simulink model "feedbacksInGuyton72"  (R2018a)
settings: Solver=VariableStepAuto  StartTime=0.0  StopTime=inf  RelTol=1e-3
settings Model: Creator=Jirka  LastModifiedBy=Jirka

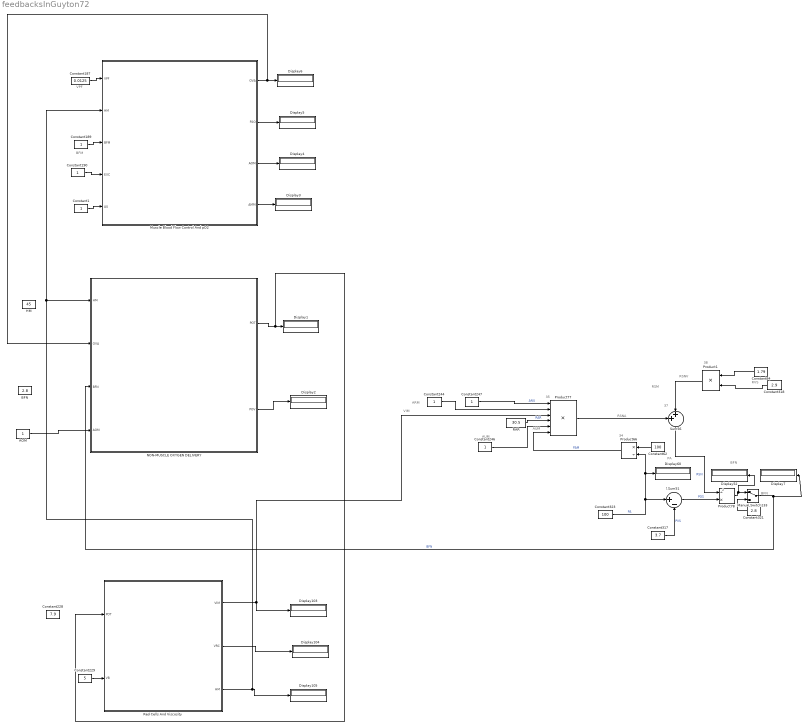
== system feedbacksInGuyton72 ==
  note: VPF
  note: BFM
  note: AUM
  note: ARM
  note: BFN
  note: VIM
  note: AUM
  note: RSM
  note: 1
  note: 35
  note: RSNV
  note: 37
  note: 2
  note: BFN
  note: PA
  note: 34
  note: RSNA
  note: RVS
  note: 38
  AOM : Constant
  BFN : Constant  Value=2.8
  Constant{1,189..190,244,246..247} (6 alike) : Constant
  Constant187 : Constant  Value=0.0125
  Constant228 : Constant  Value=7.9
  Constant229 : Constant  Value=5
  Constant317 : Constant  Value=3.7
  Constant318 : Constant  Value=2.9
  Constant321 : Constant  Value=2.8
  Constant323 : Constant  Value=100
  Constant62 : Constant  Value=100
  Constant84 : Constant  Value=1.79
  Display{1..7,52,60,103..105} (12 alike) : Display
  HM : Constant  Value=45
  Manual Switch133 : ManualSwitch
  Muscle Blood Flow Control And pO2 : Subsystem
      settings: MinAlgLoopOccurrences=on
      mask Display: disp('MUSCLE BLOOD FLOW CONTROL AND PO2\n\nINTPUTS:\nVPF - volume of free fluid in the pulmonary interstitium \nHM - hematocrit [%]\nBFM - blood flow in muscles \n [l/min]\nEXC - Effect of excercise on the metabolic usage \nof oxygen by the muscles [ratio to resting state]\nAU - overall activity of autonomic system\n  \nOUTPUTS:\nOVA - oxygen content of arterial blood \n[ml O2 STPD/l blood] \nP2O - muscle cell PO2  [torr]\nAOM - autonomic effect on tissue oxygenation \nAMM - muscle vascular constriction caused by logical tissue control\n[multiplifier, ratio to normal]\n\n')
  NON-MUSCLE OXYGEN DELIVERY : Subsystem
      mask Display: disp('NON-MUSCLE OXYGEN DELIVERY\n\nINTPUTS:\nHM-hematocrit [%]\nOVA-oxygen volume in aortic blood [ml O2/l blood]\nBFN-blood flow in non-muscle, non-renal tissues [l/min]\nAOM-autonomic effect on tissue oxygen utilization\n\nOUTPUTS:\nPOT-non-muscle cell PO2  [torr]\nPOV-non-muscle venous PO2 [torr]\n')
  Product1 : Product  SaturateOnIntegerOverflow=on  RndMeth=Zero  InputSameDT=on  OutDataTypeStr=Inherit: Same as first input
  Product66 : Product  Inputs=*/  SaturateOnIntegerOverflow=on  RndMeth=Zero  InputSameDT=on  OutDataTypeStr=Inherit: Same as first input
  Product77 : Product  Inputs=6  SaturateOnIntegerOverflow=on  RndMeth=Zero  InputSameDT=on  OutDataTypeStr=Inherit: Same as first input
  Product78 : Product  Inputs=/*  SaturateOnIntegerOverflow=on  RndMeth=Zero  InputSameDT=on  OutDataTypeStr=Inherit: Same as first input
  RAR : Constant  Value=30.5
  Red Cells And Viscosity : Subsystem
      settings: MinAlgLoopOccurrences=on
      mask Display: disp('RED CELLS AND VISCOSITY\n\nINTPUT:\nPOT - non-muscle cell PO2 [torr]\nVB - volume of blood [l]\n\nOUTPUT:\nVIM - blood viscosity [ratio to normal]\nHM - hematocrit [%]\nVRC - volume of red blood cells []\n')
  Sum51 : Sum  Inputs=|+-  SaturateOnIntegerOverflow=on  InputSameDT=on  OutDataTypeStr=Inherit: Same as first input
  Sum56 : Sum  Inputs=++|  SaturateOnIntegerOverflow=on  InputSameDT=on  OutDataTypeStr=Inherit: Same as first input
  wires:
  Constant229/1 -> Red Cells And Viscosity/2(VB)
  Red Cells And Viscosity/2(VRC) -> Display104/1
  AOM/1 -> NON-MUSCLE OXYGEN DELIVERY/4(AOM)
  NON-MUSCLE OXYGEN DELIVERY/2(POV) -> Display2/1
  Muscle Blood Flow Control And pO2/2(P2O) -> Display5/1
  Muscle Blood Flow Control And pO2/3(AOM) -> Display4/1
  Muscle Blood Flow Control And pO2/4(AMM) -> Display3/1
  Constant190/1 -> Muscle Blood Flow Control And pO2/4(EXC)
  Constant189/1 -> Muscle Blood Flow Control And pO2/3(BFM)
  Constant187/1 -> Muscle Blood Flow Control And pO2/1(VPF)
  Constant1/1 -> Muscle Blood Flow Control And pO2/5(AU)
  Muscle Blood Flow Control And pO2/1(OVA) -> NON-MUSCLE OXYGEN DELIVERY/2(OVA), Display6/1
  NON-MUSCLE OXYGEN DELIVERY/1(POT) -> Red Cells And Viscosity/1(POT), Display1/1
  Red Cells And Viscosity/3(HM) -> Muscle Blood Flow Control And pO2/2(HM), NON-MUSCLE OXYGEN DELIVERY/1(HM), Display105/1
  Sum56/1 -> Product78/1  "RSN"
  Red Cells And Viscosity/1(VIM) -> Display103/1, Product77/3
  Constant247/1 -> Product77/1  "ANU"
  Product1/1 -> Sum56/2
  Manual Switch133/1 -> Display7/1, NON-MUSCLE OXYGEN DELIVERY/3(BFN)  "BFN"
  Sum51/1 -> Product78/2  "PGS"
  Product66/1 -> Product77/6  "PAM"
  Constant62/1 -> Product66/1
  Product77/1 -> Sum56/1
  Constant246/1 -> Product77/5
  Constant244/1 -> Product77/2
  Constant323/1 -> Sum51/1, Display60/1, Product66/2  "PA"
  RAR/1 -> Product77/4  "RAR"
  Constant321/1 -> Manual Switch133/2
  Product78/1 -> Display52/1, Manual Switch133/1
  Constant84/1 -> Product1/1
  Constant318/1 -> Product1/2
  Constant317/1 -> Sum51/2  "PVS"

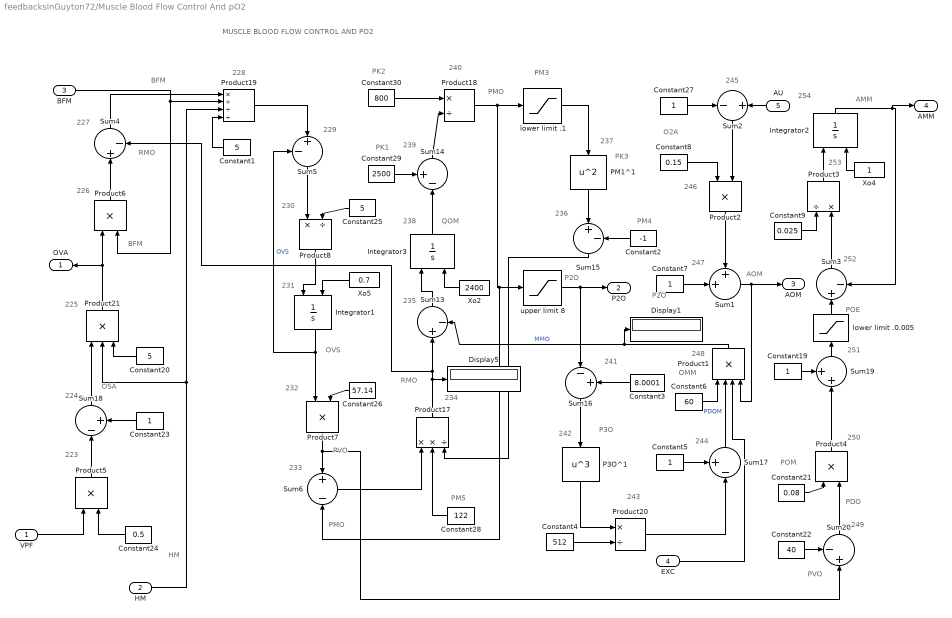
== system feedbacksInGuyton72/Muscle Blood Flow Control And pO2 ==
  note: PM5
  note: POM
  note: 244
  note: AMM
  note: 249
  note: PM3
  note: POE
  note: PK1
  note: RMO
  note: 251
  note: 236
  note: 254
  note: 240
  note: 245
  note: P2O
  note: 250
  note: P2O
  note: 252
  note: PMO
  note: OSA
  note: 253
  note: PM4
  note: PDO
  note: 247
  note: 237
  note: 239
  note: PK3
  note: PMO
  note: 246
  note: RMO
  note: BFM
  note: 243
  note: 242
  note: BFM
  note: PVO
  note: HM
  note: AOM
  note: OMM
  note: MUSCLE BLOOD FLOW CONTROL AND PO2
  note: 223
  note: 229
  note: 235
  note: 232
  note: O2A
  note: 227
  note: QOM
  note: 241
  note: PVO
  note: 228
  note: 248
  note: 226
  note: 225
  note: 231
  note: OVS
  note: 230
  note: 238
  note: P3O
  note: 234
  note: 224
  note: 233
  note: PK2
  VPF : Inport
  HM : Inport  Port=2
  BFM : Inport  Port=3
  EXC : Inport  Port=4
  AU : Inport  Port=5
  Constant1 : Constant  Value=5
  Constant{5,7,19,23,27} (5 alike) : Constant
  Constant2 : Constant  Value=-1
  Constant20 : Constant  Value=5
  Constant21 : Constant  Value=0.08
  Constant22 : Constant  Value=40
  Constant24 : Constant  Value=0.5
  Constant25 : Constant  Value=5
  Constant26 : Constant  Value=57.14
  Constant28 : Constant  Value=122
  Constant29 : Constant  Value=2500
  Constant3 : Constant  Value=8.0001
  Constant30 : Constant  Value=800
  Constant4 : Constant  Value=512
  Constant6 : Constant  Value=60
  Constant8 : Constant  Value=0.15
  Constant9 : Constant  Value=0.025
  Display1 : Display
  Display5 : Display
  Integrator1 : Integrator  InitialConditionSource=external
  Integrator2 : Integrator  InitialConditionSource=external  InitialCondition=2399.9633789
  Integrator3 : Integrator  InitialConditionSource=external  InitialCondition=2399.9633789
  P3O^1 : Fcn  Expr=u^3
  PM1^1 : Fcn  Expr=u^2
  Product1 : Product  Inputs=4  SaturateOnIntegerOverflow=on  RndMeth=Zero  InputSameDT=on  OutDataTypeStr=Inherit: Same as first input
  Product17 : Product  Inputs=**/  SaturateOnIntegerOverflow=on  RndMeth=Zero  InputSameDT=on  OutDataTypeStr=Inherit: Same as first input
  Product18 : Product  Inputs=*/  SaturateOnIntegerOverflow=on  RndMeth=Zero  InputSameDT=on  OutDataTypeStr=Inherit: Same as first input
  Product19 : Product  Inputs=*///  SaturateOnIntegerOverflow=on  RndMeth=Zero  InputSameDT=on  OutDataTypeStr=Inherit: Same as first input
  Product{2,4..7} (5 alike) : Product  SaturateOnIntegerOverflow=on  RndMeth=Zero  InputSameDT=on  OutDataTypeStr=Inherit: Same as first input
  Product20 : Product  Inputs=*/  SaturateOnIntegerOverflow=on  RndMeth=Zero  InputSameDT=on  OutDataTypeStr=Inherit: Same as first input
  Product21 : Product  Inputs=3  SaturateOnIntegerOverflow=on  RndMeth=Zero  InputSameDT=on  OutDataTypeStr=Inherit: Same as first input
  Product3 : Product  Inputs=/*  SaturateOnIntegerOverflow=on  RndMeth=Zero  InputSameDT=on  OutDataTypeStr=Inherit: Same as first input
  Product8 : Product  Inputs=*/  SaturateOnIntegerOverflow=on  RndMeth=Zero  InputSameDT=on  OutDataTypeStr=Inherit: Same as first input
  Sum1 : Sum  Inputs=++|  SaturateOnIntegerOverflow=on  InputSameDT=on  OutDataTypeStr=Inherit: Same as first input
  Sum{3..4,13,15} (4 alike) : Sum  Inputs=|+-  SaturateOnIntegerOverflow=on  InputSameDT=on  OutDataTypeStr=Inherit: Same as first input
  Sum14 : Sum  Inputs=+-|  SaturateOnIntegerOverflow=on  InputSameDT=on  OutDataTypeStr=Inherit: Same as first input
  Sum16 : Sum  Inputs=|-+  SaturateOnIntegerOverflow=on  InputSameDT=on  OutDataTypeStr=Inherit: Same as first input
  Sum17 : Sum  Inputs=+-|  SaturateOnIntegerOverflow=on  InputSameDT=on  OutDataTypeStr=Inherit: Same as first input
  Sum18 : Sum  Inputs=|-+  SaturateOnIntegerOverflow=on  InputSameDT=on  OutDataTypeStr=Inherit: Same as first input
  Sum19 : Sum  Inputs=++|  SaturateOnIntegerOverflow=on  InputSameDT=on  OutDataTypeStr=Inherit: Same as first input
  Sum2 : Sum  Inputs=-|+  SaturateOnIntegerOverflow=on  InputSameDT=on  OutDataTypeStr=Inherit: Same as first input
  Sum20 : Sum  Inputs=-+|  SaturateOnIntegerOverflow=on  InputSameDT=on  OutDataTypeStr=Inherit: Same as first input
  Sum5 : Sum  Inputs=-+|  SaturateOnIntegerOverflow=on  InputSameDT=on  OutDataTypeStr=Inherit: Same as first input
  Sum6 : Sum  Inputs=+|-  SaturateOnIntegerOverflow=on  InputSameDT=on  OutDataTypeStr=Inherit: Same as first input
  Xo2 : Constant  Value=2400  VectorParams1D=off
  Xo4 : Constant  VectorParams1D=off
  Xo5 : Constant  Value=0.7  VectorParams1D=off
  lower limit .0.005 : Saturate  UpperLimit=inf  LowerLimit=0.005  LinearizeAsGain=off
  lower limit .1 : Saturate  UpperLimit=inf  LowerLimit=0.001  LinearizeAsGain=off
  "upper limit 8 " : Saturate  UpperLimit=8  LowerLimit=0  LinearizeAsGain=off
  OVA : Outport
  P2O : Outport  Port=2
  AOM : Outport  Port=3
  AMM : Outport  Port=4
  wires:
  Constant1/1 -> Product19/4
  PM1^1/1 -> Sum15/1
  Product2/1 -> Sum1/1
  Integrator2/1 -> AMM/1, Sum3/2
  Sum13/1 -> Integrator3/1
  Constant4/1 -> Product20/2
  Constant28/1 -> Product17/2
  Constant25/1 -> Product8/2
  Sum17/1 -> Product1/2  "PDOM"
  Product1/1 -> Display1/1, Sum13/2  "MMO"
  Product5/1 -> Sum18/1
  Constant27/1 -> Sum2/1
  Constant2/1 -> Sum15/2
  Sum16/1 -> P3O^1/1
  Constant29/1 -> Sum14/1
  Product21/1 -> OVA/1, Product6/1
  Sum20/1 -> Product4/2
  Constant24/1 -> Product5/2
  Xo4/1 -> Integrator2/2
  Constant21/1 -> Product4/1
  Constant30/1 -> Product18/1
  Xo2/1 -> Integrator3/2
  Sum15/1 -> Product17/3
  lower limit .0.005/1 -> Sum3/1
  Constant8/1 -> Product2/1
  Product4/1 -> Sum19/2
  Constant19/1 -> Sum19/1
  P3O^1/1 -> Product20/1
  Product18/1 -> lower limit .1/1, Sum6/2, "upper limit 8 "/1
  Sum2/1 -> Product2/2
  Product17/1 -> Display5/1, Sum4/2, Sum13/1
  Constant3/1 -> Sum16/2
  Product20/1 -> Sum17/2
  Constant9/1 -> Product3/1
  Constant6/1 -> Product1/1
  Constant5/1 -> Sum17/1
  Sum3/1 -> Product3/2
  Integrator3/1 -> Sum14/2
  Product3/1 -> Integrator2/1
  Sum5/1 -> Product8/1
  Product19/1 -> Sum5/2
  Sum1/1 -> AOM/1, Product1/4
  Constant26/1 -> Product7/2
  Sum6/1 -> Product17/1
  Product7/1 -> Sum6/1, Sum20/2
  Sum18/1 -> Product21/1
  Xo5/1 -> Integrator1/2
  Product8/1 -> Integrator1/1
  Sum14/1 -> Product18/2
  Integrator1/1 -> Sum5/1, Product7/1  "OVS"
  Constant7/1 -> Sum1/2
  Constant23/1 -> Sum18/2
  Product6/1 -> Sum4/1
  lower limit .1/1 -> PM1^1/1
  Constant22/1 -> Sum20/1
  "upper limit 8 "/1 -> P2O/1, Sum16/1
  Sum19/1 -> lower limit .0.005/1
  Sum4/1 -> Product19/1
  Constant20/1 -> Product21/3
  VPF/1 -> Product5/1
  EXC/1 -> Product1/3
  AU/1 -> Sum2/2
  BFM/1 -> Product6/2, Product19/2
  HM/1 -> Product19/3, Product21/2

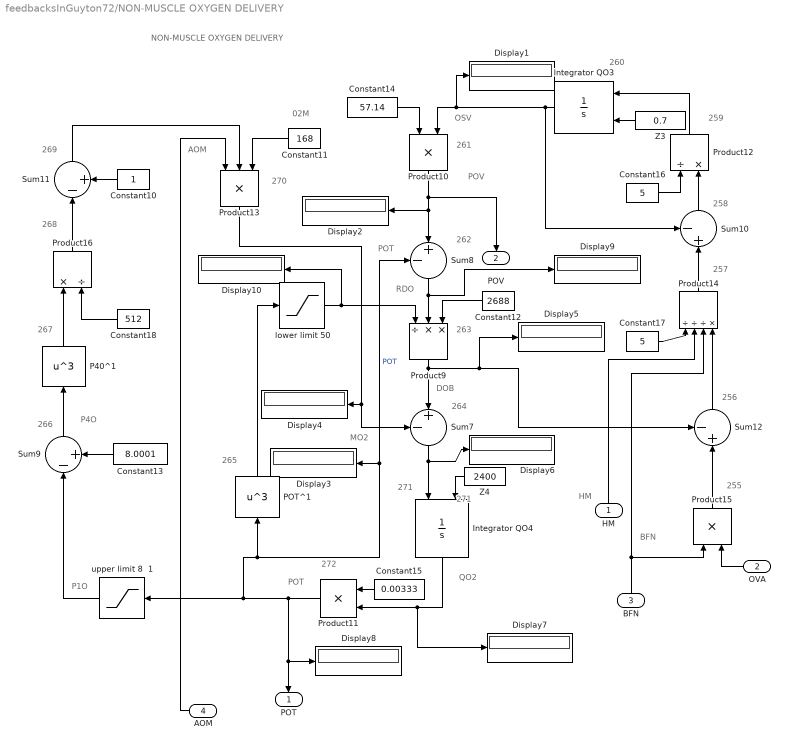
== system feedbacksInGuyton72/NON-MUSCLE OXYGEN DELIVERY ==
  note: 269
  note: 260
  note: 268
  note: 264
  note: BFN
  note: 267
  note: 259
  note: 270
  note: HM
  note: 271
  note: 257
  note: 258
  note: 261
  note: NON-MUSCLE OXYGEN DELIVERY
  note: 262
  note: 266
  note: 263
  note: 272
  note: 256
  note: 255
  note: POV
  note: OSV
  note: POT
  note: RDO
  note: DOB
  note: P1O
  note: 02M
  note: P4O
  note: MO2
  note: 265
  note: QO2
  note: 271
  note: AOM
  note: POT
  HM : Inport
  OVA : Inport  Port=2
  BFN : Inport  Port=3
  AOM : Inport  Port=4
  Constant10 : Constant
  Constant11 : Constant  Value=168
  Constant12 : Constant  Value=2688
  Constant13 : Constant  Value=8.0001
  Constant14 : Constant  Value=57.14
  Constant15 : Constant  Value=0.00333
  Constant16 : Constant  Value=5
  Constant17 : Constant  Value=5
  Constant18 : Constant  Value=512
  Display{1..10} (10 alike) : Display
  Integrator QO3 : Integrator  InitialConditionSource=external  InitialCondition=2403.143066
  Integrator QO4 : Integrator  InitialConditionSource=external  InitialCondition=2403.143066
  P40^1 : Fcn  Expr=u^3
  POT^1 : Fcn  Expr=u^3
  Product10 : Product  SaturateOnIntegerOverflow=on  RndMeth=Zero  InputSameDT=on  OutDataTypeStr=Inherit: Same as first input
  Product11 : Product  SaturateOnIntegerOverflow=on  RndMeth=Zero  InputSameDT=on  OutDataTypeStr=Inherit: Same as first input
  Product12 : Product  Inputs=/*  SaturateOnIntegerOverflow=on  RndMeth=Zero  InputSameDT=on  OutDataTypeStr=Inherit: Same as first input
  Product13 : Product  Inputs=3  SaturateOnIntegerOverflow=on  RndMeth=Zero  InputSameDT=on  OutDataTypeStr=Inherit: Same as first input
  Product14 : Product  Inputs=///*  SaturateOnIntegerOverflow=on  RndMeth=Zero  InputSameDT=on  OutDataTypeStr=Inherit: Same as first input
  Product15 : Product  SaturateOnIntegerOverflow=on  RndMeth=Zero  InputSameDT=on  OutDataTypeStr=Inherit: Same as first input
  Product16 : Product  Inputs=*/  SaturateOnIntegerOverflow=on  RndMeth=Zero  InputSameDT=on  OutDataTypeStr=Inherit: Same as first input
  Product9 : Product  Inputs=/**  SaturateOnIntegerOverflow=on  RndMeth=Zero  InputSameDT=on  OutDataTypeStr=Inherit: Same as first input
  Sum{7..8,10,12} (4 alike) : Sum  Inputs=-+|  SaturateOnIntegerOverflow=on  InputSameDT=on  OutDataTypeStr=Inherit: Same as first input
  Sum11 : Sum  Inputs=|-+  SaturateOnIntegerOverflow=on  InputSameDT=on  OutDataTypeStr=Inherit: Same as first input
  Sum9 : Sum  Inputs=|-+  SaturateOnIntegerOverflow=on  InputSameDT=on  OutDataTypeStr=Inherit: Same as first input
  Z3 : Constant  Value=0.7
  Z4 : Constant  Value=2400
  lower limit 50 : Saturate  UpperLimit=inf  LowerLimit=50  LinearizeAsGain=off
  upper limit 8  1 : Saturate  UpperLimit=8  LowerLimit=-inf  LinearizeAsGain=off  ZeroCross=off
  POT : Outport
  POV : Outport  Port=2
  wires:
  Integrator QO3/1 -> Sum10/1, Display1/1, Product10/2
  Sum12/1 -> Product14/4
  Product11/1 -> Display8/1, POT/1, POT^1/1, Display3/1, Sum8/1, upper limit 8  1/1  "POT"
  HM/1 -> Product14/2
  Product12/1 -> Integrator QO3/1
  Product10/1 -> Sum8/2, Display2/1, POV/1
  OVA/1 -> Product15/2
  Constant11/1 -> Product13/3
  Product9/1 -> Sum7/2, Display5/1, Sum12/1
  Product15/1 -> Sum12/2
  Sum7/1 -> Display6/1, Integrator QO4/1
  AOM/1 -> Product13/1
  Sum11/1 -> Product13/2
  Sum9/1 -> P40^1/1
  Z3/1 -> Integrator QO3/2
  upper limit 8  1/1 -> Sum9/1
  Constant14/1 -> Product10/1
  Sum8/1 -> Display9/1, Product9/2
  Product13/1 -> Display4/1, Sum7/1
  P40^1/1 -> Product16/1
  Constant13/1 -> Sum9/2
  Sum10/1 -> Product12/2
  Integrator QO4/1 -> Display7/1, Product11/2
  Constant10/1 -> Sum11/2
  Constant17/1 -> Product14/1
  Product16/1 -> Sum11/1
  Constant18/1 -> Product16/2
  Constant16/1 -> Product12/1
  BFN/1 -> Product15/1, Product14/3
  Product14/1 -> Sum10/2
  Z4/1 -> Integrator QO4/2
  Constant15/1 -> Product11/1
  Constant12/1 -> Product9/3
  POT^1/1 -> lower limit 50/1
  lower limit 50/1 -> Display10/1, Product9/1

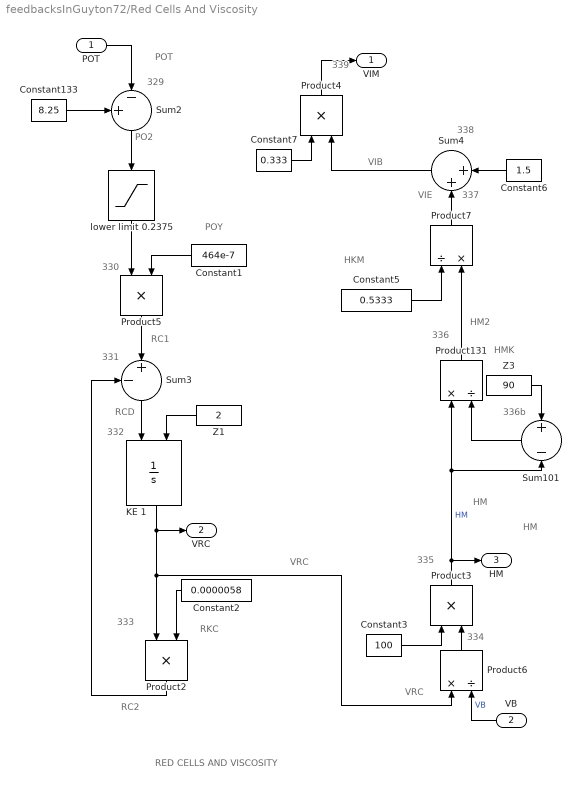
== system feedbacksInGuyton72/Red Cells And Viscosity ==
  note: HKM
  note: 336
  note: HMK
  note: HM
  note: 336b
  note: VIB
  note: HM2
  note: RKC
  note: RED CELLS AND VISCOSITY
  note: 329
  note: HM
  note: PO2
  note: 332
  note: RC1
  note: 330
  note: 331
  note: VRC
  note: VRC
  note: POY
  note: RCD
  note: 334
  note: VIE
  note: RC2
  note: 339
  note: 338
  note: 333
  note: POT
  note: 337
  note: 335
  POT : Inport
  VB : Inport  Port=2
  Constant1 : Constant  Value=464e-7
  Constant133 : Constant  Value=8.25
  Constant2 : Constant  Value=0.0000058
  Constant3 : Constant  Value=100
  Constant5 : Constant  Value=0.5333
  Constant6 : Constant  Value=1.5
  Constant7 : Constant  Value=0.333
  KE 1 : Integrator  InitialConditionSource=external  InitialCondition=74.7024
  Product131 : Product  Inputs=*/  SaturateOnIntegerOverflow=on  RndMeth=Zero  InputSameDT=on  OutDataTypeStr=Inherit: Same as first input
  Product{2..5} (4 alike) : Product  SaturateOnIntegerOverflow=on  RndMeth=Zero  InputSameDT=on  OutDataTypeStr=Inherit: Same as first input
  Product6 : Product  Inputs=*/  SaturateOnIntegerOverflow=on  RndMeth=Zero  InputSameDT=on  OutDataTypeStr=Inherit: Same as first input
  Product7 : Product  Inputs=/*  SaturateOnIntegerOverflow=on  RndMeth=Zero  InputSameDT=on  OutDataTypeStr=Inherit: Same as first input
  Sum101 : Sum  Inputs=+-  SaturateOnIntegerOverflow=on  InputSameDT=on  OutDataTypeStr=Inherit: Same as first input
  Sum2 : Sum  Inputs=+-|  SaturateOnIntegerOverflow=on  InputSameDT=on  OutDataTypeStr=Inherit: Same as first input
  Sum3 : Sum  Inputs=-+|  SaturateOnIntegerOverflow=on  InputSameDT=on  OutDataTypeStr=Inherit: Same as first input
  Sum4 : Sum  Inputs=|++  SaturateOnIntegerOverflow=on  InputSameDT=on  OutDataTypeStr=Inherit: Same as first input
  Z1 : Constant  Value=2
  Z3 : Constant  Value=90
  lower limit 0.2375 : Saturate  UpperLimit=inf  LowerLimit=0.2375  LinearizeAsGain=off
  VIM : Outport
  VRC : Outport  Port=2
  HM : Outport  Port=3
  wires:
  Sum101/1 -> Product131/2
  Z3/1 -> Sum101/1
  Product6/1 -> Product3/2
  Product2/1 -> Sum3/1
  Constant6/1 -> Sum4/1
  POT/1 -> Sum2/2
  Sum3/1 -> KE 1/1
  Constant7/1 -> Product4/1
  Product131/1 -> Product7/2
  Constant2/1 -> Product2/2
  Product5/1 -> Sum3/2
  Product7/1 -> Sum4/2
  Product3/1 -> HM/1, Sum101/2, Product131/1  "HM"
  Sum4/1 -> Product4/2
  Sum2/1 -> lower limit 0.2375/1
  Constant5/1 -> Product7/1
  Constant1/1 -> Product5/2
  Constant3/1 -> Product3/1
  lower limit 0.2375/1 -> Product5/1
  Z1/1 -> KE 1/2
  KE 1/1 -> VRC/1, Product2/1, Product6/1
  VB/1 -> Product6/2  "VB"
  Product4/1 -> VIM/1
  Constant133/1 -> Sum2/1
